simulink subsystem "GenericLFO"  (R2024a)
settings: Solver=VariableStepAuto  StartTime=0.0  StopTime=10.0  RelTol=1e-3
model mask{wave_len=16384, max_freq=20}
libraries: simulink x1
settings Model: Creator=dfurodet  LastModifiedBy=dfurodet

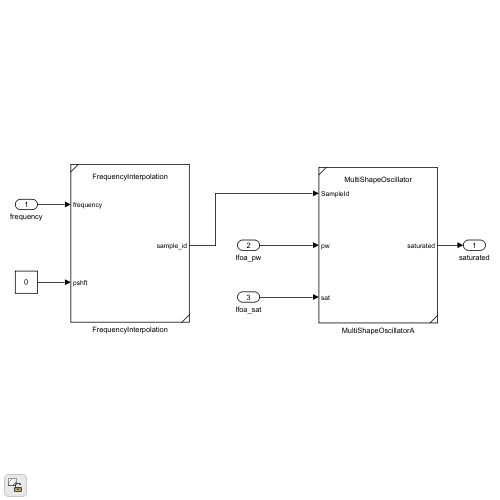
[thumbnail: Simulink's stored preview of the top-level diagram]
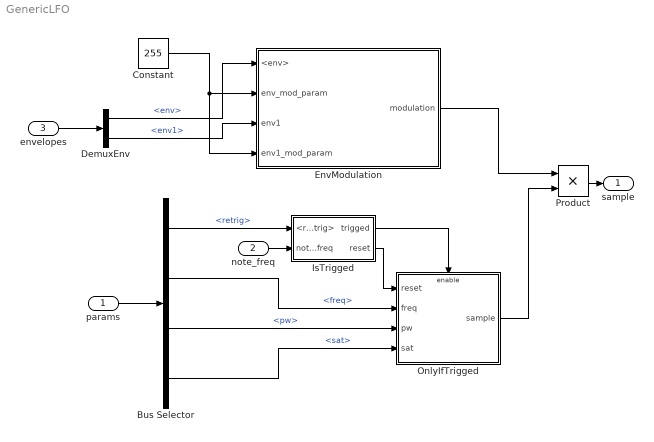
== system GenericLFO ==
  params : Inport
  note_freq : Inport  Port=2
  envelopes : Inport  Port=3
  Bus Selector : BusSelector  OutputSignals=retrig,freq,pw,sat
  Constant : Constant  Value=255  OutDataTypeStr=uint8
  DemuxEnv : BusSelector  OutputSignals=env,env1
  EnvModulation : Subsystem
  IsTrigged : Subsystem
  OnlyIfTrigged : Subsystem  TreatAsAtomicUnit=on
  Product : Product
  sample : Outport
  wires:
  params/1 -> Bus Selector/1
  Bus Selector/2 -> OnlyIfTrigged/2(freq)  "<freq>"
  Bus Selector/3 -> OnlyIfTrigged/3(pw)  "<pw>"
  Bus Selector/4 -> OnlyIfTrigged/4(sat)  "<sat>"
  Bus Selector/1 -> IsTrigged/1(<retrig>)  "<retrig>"
  note_freq/1 -> IsTrigged/2(note_freq)
  IsTrigged/1(trigged) -> OnlyIfTrigged/Enable
  IsTrigged/2(reset) -> OnlyIfTrigged/1(reset)
  envelopes/1 -> DemuxEnv/1
  DemuxEnv/1 -> EnvModulation/1(<env>)  "<env>"
  Constant/1 -> EnvModulation/2(env_mod_param), EnvModulation/4(env1_mod_param)
  EnvModulation/1(modulation) -> Product/1
  OnlyIfTrigged/1(sample) -> Product/2
  Product/1 -> sample/1
  DemuxEnv/2 -> EnvModulation/3(env1)  "<env1>"

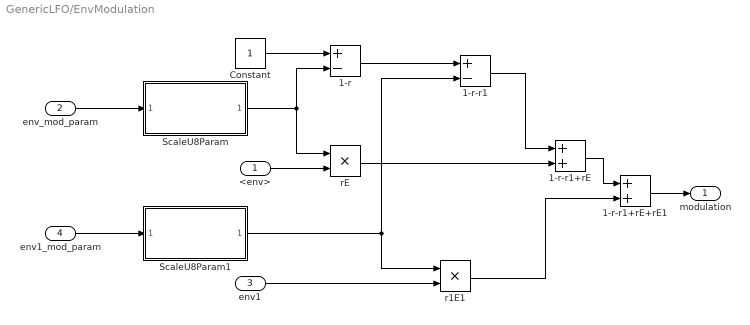
== system GenericLFO/EnvModulation ==
  <env> : Inport
  env_mod_param : Inport  Port=2
  env1 : Inport  Port=3
  env1_mod_param : Inport  Port=4
  1-r : Sum  Inputs=+-
  1-r-r1 : Sum  Inputs=+-
  1-r-r1+rE : Sum
  1-r-r1+rE+rE1 : Sum
  Constant : Constant
  ScaleU8Param : Subsystem  ReferencedSubsystem=ScaleU8Param
  ScaleU8Param1 : Subsystem  ReferencedSubsystem=ScaleU8Param
  r1E1 : Product
  rE : Product
  modulation : Outport
  wires:
  env_mod_param/1 -> ScaleU8Param/1
  ScaleU8Param/1 -> 1-r/2, rE/1
  1-r-r1+rE+rE1/1 -> modulation/1
  r1E1/1 -> 1-r-r1+rE+rE1/2
  1-r-r1+rE/1 -> 1-r-r1+rE+rE1/1
  env1/1 -> r1E1/2
  ScaleU8Param1/1 -> 1-r-r1/2, r1E1/1
  1-r-r1/1 -> 1-r-r1+rE/1
  1-r/1 -> 1-r-r1/1
  env1_mod_param/1 -> ScaleU8Param1/1
  <env>/1 -> rE/2
  rE/1 -> 1-r-r1+rE/2
  Constant/1 -> 1-r/1

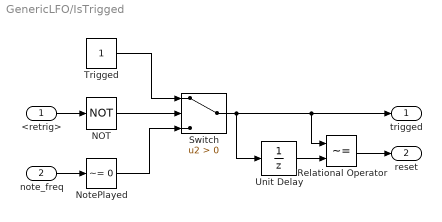
== system GenericLFO/IsTrigged ==
  <retrig> : Inport
  note_freq : Inport  Port=2
  NOT : Logic  Operator=NOT  IconShape=distinctive  AllPortsSameDT=off  OutDataTypeStr=boolean
  NotePlayed : simulink/Logic and Bit Operations/Compare To Zero  relop=~=  OutDataTypeStr=boolean
  Relational Operator : RelationalOperator  Operator=~=  OutDataTypeStr=boolean  RndMeth=Simplest  InputSameDT=off
  Switch : Switch  Criteria=u2 > Threshold  SaturateOnIntegerOverflow=off  InputSameDT=off
  Trigged : Constant  OutDataTypeStr=boolean
  Unit Delay : UnitDelay  SampleTime=-1  HasFrameUpgradeWarning=on
  trigged : Outport
  reset : Outport  Port=2
  wires:
  Relational Operator/1 -> reset/1
  Unit Delay/1 -> Relational Operator/2
  NOT/1 -> Switch/2
  note_freq/1 -> NotePlayed/1
  NotePlayed/1 -> Switch/3
  Trigged/1 -> Switch/1
  <retrig>/1 -> NOT/1
  Switch/1 -> Unit Delay/1, trigged/1, Relational Operator/1

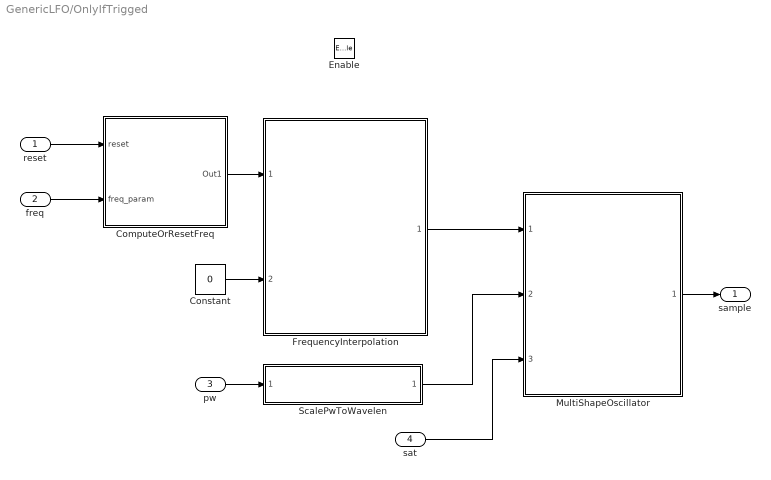
== system GenericLFO/OnlyIfTrigged ==
  reset : Inport
  freq : Inport  Port=2
  pw : Inport  Port=3
  sat : Inport  Port=4
  Enable : EnablePort
  ComputeOrResetFreq : Subsystem
  Constant : Constant  Value=0
  FrequencyInterpolation : Subsystem  ReferencedSubsystem=FrequencyInterpolation
  MultiShapeOscillator : Subsystem  ReferencedSubsystem=MultiShapeOscillator
  ScalePwToWavelen : Subsystem  ReferencedSubsystem=ScaleParamToWavelen
  sample : Outport
  wires:
  ComputeOrResetFreq/1(Out1) -> FrequencyInterpolation/1
  freq/1 -> ComputeOrResetFreq/2(freq_param)
  reset/1 -> ComputeOrResetFreq/1(reset)
  MultiShapeOscillator/1 -> sample/1
  sat/1 -> MultiShapeOscillator/3
  ScalePwToWavelen/1 -> MultiShapeOscillator/2
  FrequencyInterpolation/1 -> MultiShapeOscillator/1
  pw/1 -> ScalePwToWavelen/1
  Constant/1 -> FrequencyInterpolation/2

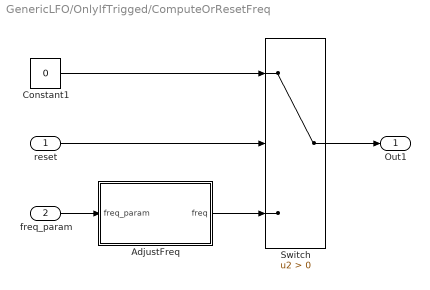
== system GenericLFO/OnlyIfTrigged/ComputeOrResetFreq ==
  reset : Inport
  freq_param : Inport  Port=2
  AdjustFreq : Subsystem
  Constant1 : Constant  Value=0
  Switch : Switch  Criteria=u2 > Threshold  SaturateOnIntegerOverflow=off  InputSameDT=off
  Out1 : Outport
  wires:
  Switch/1 -> Out1/1
  freq_param/1 -> AdjustFreq/1(freq_param)
  reset/1 -> Switch/2
  AdjustFreq/1(freq) -> Switch/3
  Constant1/1 -> Switch/1

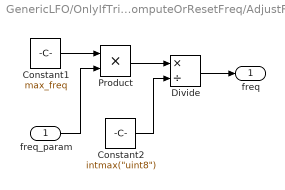
== system GenericLFO/OnlyIfTrigged/ComputeOrResetFreq/AdjustFreq ==
  freq_param : Inport
  Constant1 : Constant  Value=max_freq
  Constant2 : Constant  Value="intmax(\"uint8\")"
  Divide : Product  Inputs=*/
  Product : Product
  freq : Outport
  wires:
  Divide/1 -> freq/1
  freq_param/1 -> Product/2
  Constant2/1 -> Divide/2
  Constant1/1 -> Product/1
  Product/1 -> Divide/1
